simulink model "Plant"  (R2019a)
settings: Solver=FixedStepDiscrete  StartTime=0.0  StopTime=40  FixedStep=0.25  RelTol=1e-3
settings Model: Creator=Athar Hussain  LastModifiedBy=Athar Hussain

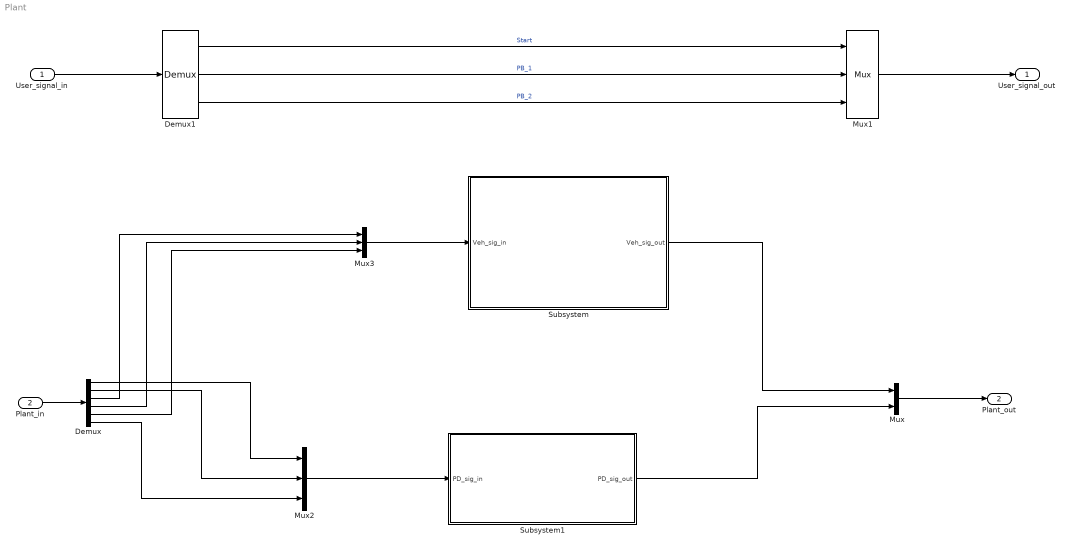
== system Plant ==
  User_signal_in : Inport
  Plant_in : Inport  Port=2
  Demux : Demux  Outputs=6
  Demux1 : Demux  Outputs=3
  Mux : Mux  Inputs=2
  Mux1 : Mux  Inputs=3
  Mux2 : Mux  Inputs=3
  Mux3 : Mux  Inputs=3
  Subsystem : Subsystem
  Subsystem1 : Subsystem
  User_signal_out : Outport
  Plant_out : Outport  Port=2
  wires:
  Subsystem/1(Veh_sig_out) -> Mux/1
  Plant_in/1 -> Demux/1
  Subsystem1/1(PD_sig_out) -> Mux/2
  Mux/1 -> Plant_out/1
  Mux1/1 -> User_signal_out/1
  User_signal_in/1 -> Demux1/1
  Demux/1 -> Mux2/1
  Demux/2 -> Mux2/2
  Demux/6 -> Mux2/3
  Demux/3 -> Mux3/1
  Demux/4 -> Mux3/2
  Demux/5 -> Mux3/3
  Mux3/1 -> Subsystem/1(Veh_sig_in)
  Mux2/1 -> Subsystem1/1(PD_sig_in)
  Demux1/1 -> Mux1/1  "Start"
  Demux1/2 -> Mux1/2  "PB_1"
  Demux1/3 -> Mux1/3  "PB_2"

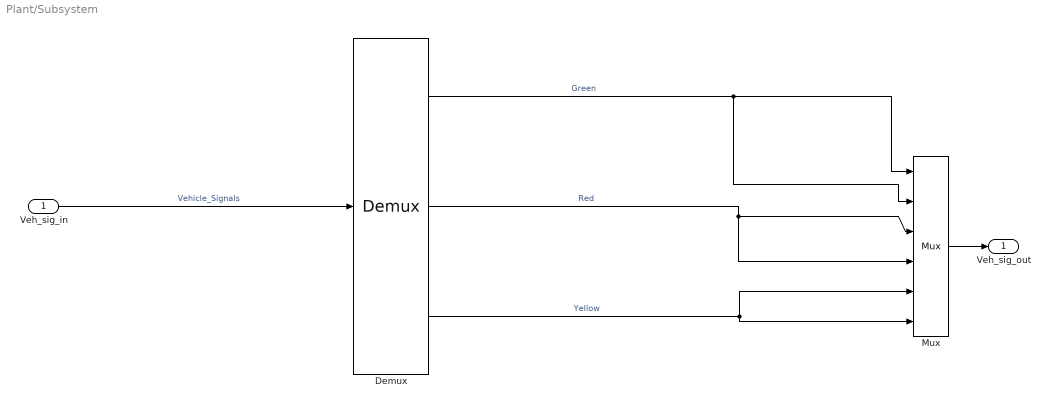
== system Plant/Subsystem ==
  Veh_sig_in : Inport
  Demux : Demux  Outputs=3
  Mux : Mux  Inputs=6
  Veh_sig_out : Outport
  wires:
  Demux/2 -> Mux/3, Mux/4  "Red"
  Demux/1 -> Mux/1, Mux/2  "Green"
  Demux/3 -> Mux/6, Mux/5  "Yellow"
  Veh_sig_in/1 -> Demux/1  "Vehicle_Signals"
  Mux/1 -> Veh_sig_out/1

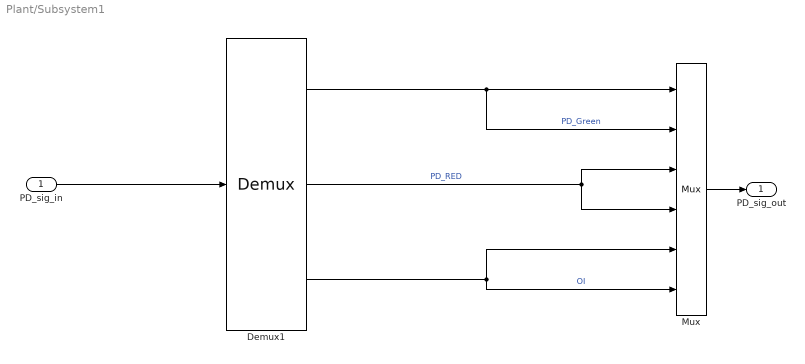
== system Plant/Subsystem1 ==
  PD_sig_in : Inport
  Demux1 : Demux  Outputs=3
  Mux : Mux  Inputs=6
  PD_sig_out : Outport
  wires:
  Demux1/1 -> Mux/1, Mux/2  "PD_Green"
  Demux1/2 -> Mux/4, Mux/3  "PD_RED"
  Demux1/3 -> Mux/6, Mux/5  "OI"
  PD_sig_in/1 -> Demux1/1
  Mux/1 -> PD_sig_out/1
